simulink library "tp333079"  (Simulink 5.0)
values from neighbouring files (symbols this model uses):
  b = 1    [main_flock3.m]    (also in main_flock4.m; params_flocking_ros.m)
undefined symbols (not defined in the file or in its folder): AC, AlphaBnd, BetaBnd, CDda, CDde, CDdf, CDdr, CDM, CDmin, CGempty, CGgross, CL0, CLa, CLalphadot, Clbeta, Clda, CLde, CLdf, Cldr, CLM, CLmind, Clp, CLq, Clr, Cm0, Cma, Cmalphadot, Cmde, Cmdf, CmM, Cmq, Cnbeta, Cnda, Cndr, Cnp, Cnr, CP, CT, CYbeta, CYda, CYdr, CYp, CYr, Displacement, dmy, Engine, EulerIni, FuelFlow, FuelIni, J, Jempty, Jeng, Jgross, Jprop, MAC, MAP, MAPLim, MassIni, MaxPower, mempty ... (+26)
libraries: aerosimlib x325, simulink3 x42
(part 11 of 11)

== system tp333079/FlightGear-Compatible/Complete Aircraft/CESSNA-172/Aerodynamics/Roll/Cl aileron ==
  RowParam : Inport  Port=1  PortDimensions=-1  SampleTime=-1  DataType=auto
      settings: SignalType=auto
  ColParam : Inport  Port=2  PortDimensions=-1  SampleTime=-1  DataType=auto
      settings: SignalType=auto
  Value : aerosimlib/FlightGear-Compatible/Aerodynamics/Value  Value=AC.Aerodynamics.Roll.ClDa
  term2 : Terminator
  Coeff : Outport  Port=1
  wires:
  RowParam/1 -> Value/1
  Value/1 -> Coeff/1
  ColParam/1 -> term2/1

== system tp333079/FlightGear-Compatible/Complete Aircraft/CESSNA-172/Aerodynamics/Roll/Cl beta ==
  RowParam : Inport  Port=1  PortDimensions=-1  SampleTime=-1  DataType=auto
      settings: SignalType=auto
  ColParam : Inport  Port=2  PortDimensions=-1  SampleTime=-1  DataType=auto
      settings: SignalType=auto
  Vector : aerosimlib/FlightGear-Compatible/Aerodynamics/Vector  Vector=AC.Aerodynamics.Roll.Clb
  term2 : Terminator
  Coeff : Outport  Port=1
  wires:
  RowParam/1 -> Vector/1
  Vector/1 -> Coeff/1
  ColParam/1 -> term2/1

== system tp333079/FlightGear-Compatible/Complete Aircraft/CESSNA-172/Aerodynamics/Roll/Cl rudder ==
  RowParam : Inport  Port=1  PortDimensions=-1  SampleTime=-1  DataType=auto
      settings: SignalType=auto
  ColParam : Inport  Port=2  PortDimensions=-1  SampleTime=-1  DataType=auto
      settings: SignalType=auto
  Value : aerosimlib/FlightGear-Compatible/Aerodynamics/Value  Value=AC.Aerodynamics.Roll.Cldr
  term2 : Terminator
  Coeff : Outport  Port=1
  wires:
  RowParam/1 -> Value/1
  Value/1 -> Coeff/1
  ColParam/1 -> term2/1

== system tp333079/FlightGear-Compatible/Complete Aircraft/CESSNA-172/Aerodynamics/Roll/Clp ==
  RowParam : Inport  Port=1  PortDimensions=-1  SampleTime=-1  DataType=auto
      settings: SignalType=auto
  ColParam : Inport  Port=2  PortDimensions=-1  SampleTime=-1  DataType=auto
      settings: SignalType=auto
  Value : aerosimlib/FlightGear-Compatible/Aerodynamics/Value  Value=AC.Aerodynamics.Roll.Clp
  term2 : Terminator
  Coeff : Outport  Port=1
  wires:
  RowParam/1 -> Value/1
  Value/1 -> Coeff/1
  ColParam/1 -> term2/1

== system tp333079/FlightGear-Compatible/Complete Aircraft/CESSNA-172/Aerodynamics/Roll/Clr ==
  RowParam : Inport  Port=1  PortDimensions=-1  SampleTime=-1  DataType=auto
      settings: SignalType=auto
  ColParam : Inport  Port=2  PortDimensions=-1  SampleTime=-1  DataType=auto
      settings: SignalType=auto
  Table : aerosimlib/FlightGear-Compatible/Aerodynamics/Table  Table=AC.Aerodynamics.Roll.Clr
  Coeff : Outport  Port=1
  wires:
  RowParam/1 -> Table/1
  ColParam/1 -> Table/2
  Table/1 -> Coeff/1

== system tp333079/FlightGear-Compatible/Complete Aircraft/CESSNA-172/Aerodynamics/Side/CY aileron ==
  RowParam : Inport  Port=1  PortDimensions=-1  SampleTime=-1  DataType=auto
      settings: SignalType=auto
  ColParam : Inport  Port=2  PortDimensions=-1  SampleTime=-1  DataType=auto
      settings: SignalType=auto
  Value : aerosimlib/FlightGear-Compatible/Aerodynamics/Value  Value=AC.Aerodynamics.Side.CYda
  term2 : Terminator
  Coeff : Outport  Port=1
  wires:
  RowParam/1 -> Value/1
  Value/1 -> Coeff/1
  ColParam/1 -> term2/1

== system tp333079/FlightGear-Compatible/Complete Aircraft/CESSNA-172/Aerodynamics/Side/CY beta ==
  RowParam : Inport  Port=1  PortDimensions=-1  SampleTime=-1  DataType=auto
      settings: SignalType=auto
  ColParam : Inport  Port=2  PortDimensions=-1  SampleTime=-1  DataType=auto
      settings: SignalType=auto
  Table : aerosimlib/FlightGear-Compatible/Aerodynamics/Table  Table=AC.Aerodynamics.Side.CYb
  Coeff : Outport  Port=1
  wires:
  RowParam/1 -> Table/1
  ColParam/1 -> Table/2
  Table/1 -> Coeff/1

== system tp333079/FlightGear-Compatible/Complete Aircraft/CESSNA-172/Aerodynamics/Side/CY rudder ==
  RowParam : Inport  Port=1  PortDimensions=-1  SampleTime=-1  DataType=auto
      settings: SignalType=auto
  ColParam : Inport  Port=2  PortDimensions=-1  SampleTime=-1  DataType=auto
      settings: SignalType=auto
  Value : aerosimlib/FlightGear-Compatible/Aerodynamics/Value  Value=AC.Aerodynamics.Side.CYdr
  term2 : Terminator
  Coeff : Outport  Port=1
  wires:
  RowParam/1 -> Value/1
  Value/1 -> Coeff/1
  ColParam/1 -> term2/1

== system tp333079/FlightGear-Compatible/Complete Aircraft/CESSNA-172/Aerodynamics/Side/CYp ==
  RowParam : Inport  Port=1  PortDimensions=-1  SampleTime=-1  DataType=auto
      settings: SignalType=auto
  ColParam : Inport  Port=2  PortDimensions=-1  SampleTime=-1  DataType=auto
      settings: SignalType=auto
  Table : aerosimlib/FlightGear-Compatible/Aerodynamics/Table  Table=AC.Aerodynamics.Side.CYp
  Coeff : Outport  Port=1
  wires:
  RowParam/1 -> Table/1
  ColParam/1 -> Table/2
  Table/1 -> Coeff/1

== system tp333079/FlightGear-Compatible/Complete Aircraft/CESSNA-172/Aerodynamics/Side/CYr ==
  RowParam : Inport  Port=1  PortDimensions=-1  SampleTime=-1  DataType=auto
      settings: SignalType=auto
  ColParam : Inport  Port=2  PortDimensions=-1  SampleTime=-1  DataType=auto
      settings: SignalType=auto
  Table : aerosimlib/FlightGear-Compatible/Aerodynamics/Table  Table=AC.Aerodynamics.Side.CYr
  Coeff : Outport  Port=1
  wires:
  RowParam/1 -> Table/1
  ColParam/1 -> Table/2
  Table/1 -> Coeff/1

== system tp333079/FlightGear-Compatible/Complete Aircraft/CESSNA-172/Aerodynamics/Yaw/Cn aileron ==
  RowParam : Inport  Port=1  PortDimensions=-1  SampleTime=-1  DataType=auto
      settings: SignalType=auto
  ColParam : Inport  Port=2  PortDimensions=-1  SampleTime=-1  DataType=auto
      settings: SignalType=auto
  Value : aerosimlib/FlightGear-Compatible/Aerodynamics/Value  Value=AC.Aerodynamics.Yaw.Cnda
  term2 : Terminator
  Coeff : Outport  Port=1
  wires:
  ColParam/1 -> term2/1
  Value/1 -> Coeff/1
  RowParam/1 -> Value/1

== system tp333079/FlightGear-Compatible/Complete Aircraft/CESSNA-172/Aerodynamics/Yaw/Cn beta ==
  RowParam : Inport  Port=1  PortDimensions=-1  SampleTime=-1  DataType=auto
      settings: SignalType=auto
  ColParam : Inport  Port=2  PortDimensions=-1  SampleTime=-1  DataType=auto
      settings: SignalType=auto
  Vector : aerosimlib/FlightGear-Compatible/Aerodynamics/Vector  Vector=AC.Aerodynamics.Yaw.Cnb
  term2 : Terminator
  Coeff : Outport  Port=1
  wires:
  ColParam/1 -> term2/1
  Vector/1 -> Coeff/1
  RowParam/1 -> Vector/1

== system tp333079/FlightGear-Compatible/Complete Aircraft/CESSNA-172/Aerodynamics/Yaw/Cn rudder ==
  RowParam : Inport  Port=1  PortDimensions=-1  SampleTime=-1  DataType=auto
      settings: SignalType=auto
  ColParam : Inport  Port=2  PortDimensions=-1  SampleTime=-1  DataType=auto
      settings: SignalType=auto
  Value : aerosimlib/FlightGear-Compatible/Aerodynamics/Value  Value=AC.Aerodynamics.Yaw.Cndr
  term2 : Terminator
  Coeff : Outport  Port=1
  wires:
  ColParam/1 -> term2/1
  Value/1 -> Coeff/1
  RowParam/1 -> Value/1

== system tp333079/FlightGear-Compatible/Complete Aircraft/CESSNA-172/Aerodynamics/Yaw/Cnp ==
  RowParam : Inport  Port=1  PortDimensions=-1  SampleTime=-1  DataType=auto
      settings: SignalType=auto
  ColParam : Inport  Port=2  PortDimensions=-1  SampleTime=-1  DataType=auto
      settings: SignalType=auto
  Value : aerosimlib/FlightGear-Compatible/Aerodynamics/Value  Value=AC.Aerodynamics.Yaw.Cnp
  term2 : Terminator
  Coeff : Outport  Port=1
  wires:
  ColParam/1 -> term2/1
  Value/1 -> Coeff/1
  RowParam/1 -> Value/1

== system tp333079/FlightGear-Compatible/Complete Aircraft/CESSNA-172/Aerodynamics/Yaw/Cnr ==
  RowParam : Inport  Port=1  PortDimensions=-1  SampleTime=-1  DataType=auto
      settings: SignalType=auto
  ColParam : Inport  Port=2  PortDimensions=-1  SampleTime=-1  DataType=auto
      settings: SignalType=auto
  Value : aerosimlib/FlightGear-Compatible/Aerodynamics/Value  Value=AC.Aerodynamics.Yaw.Cnr
  term2 : Terminator
  Coeff : Outport  Port=1
  wires:
  ColParam/1 -> term2/1
  Value/1 -> Coeff/1
  RowParam/1 -> Value/1

== system tp333079/FlightGear-Compatible/Complete Aircraft/CESSNA-182/Aerodynamics/Drag/CD alpha ==
  RowParam : Inport  Port=1  PortDimensions=-1  SampleTime=-1  DataType=auto
      settings: SignalType=auto
  ColParam : Inport  Port=2  PortDimensions=-1  SampleTime=-1  DataType=auto
      settings: SignalType=auto
  Vector : aerosimlib/FlightGear-Compatible/Aerodynamics/Vector  Vector=AC.Aerodynamics.Drag.CDalpha
  term2 : Terminator
  Coeff : Outport  Port=1
  wires:
  ColParam/1 -> term2/1
  Vector/1 -> Coeff/1
  RowParam/1 -> Vector/1

== system tp333079/FlightGear-Compatible/Complete Aircraft/CESSNA-182/Aerodynamics/Drag/CD beta ==
  RowParam : Inport  Port=1  PortDimensions=-1  SampleTime=-1  DataType=auto
      settings: SignalType=auto
  ColParam : Inport  Port=2  PortDimensions=-1  SampleTime=-1  DataType=auto
      settings: SignalType=auto
  Value : aerosimlib/FlightGear-Compatible/Aerodynamics/Value  Value=AC.Aerodynamics.Drag.CDbeta
  term2 : Terminator
  Coeff : Outport  Port=1
  wires:
  ColParam/1 -> term2/1
  Value/1 -> Coeff/1
  RowParam/1 -> Value/1

== system tp333079/FlightGear-Compatible/Complete Aircraft/CESSNA-182/Aerodynamics/Drag/CD elevator ==
  RowParam : Inport  Port=1  PortDimensions=-1  SampleTime=-1  DataType=auto
      settings: SignalType=auto
  ColParam : Inport  Port=2  PortDimensions=-1  SampleTime=-1  DataType=auto
      settings: SignalType=auto
  Value : aerosimlib/FlightGear-Compatible/Aerodynamics/Value  Value=AC.Aerodynamics.Drag.CDDe
  term2 : Terminator
  Coeff : Outport  Port=1
  wires:
  ColParam/1 -> term2/1
  Value/1 -> Coeff/1
  RowParam/1 -> Value/1

== system tp333079/FlightGear-Compatible/Complete Aircraft/CESSNA-182/Aerodynamics/Drag/CD flap ==
  RowParam : Inport  Port=1  PortDimensions=-1  SampleTime=-1  DataType=auto
      settings: SignalType=auto
  ColParam : Inport  Port=2  PortDimensions=-1  SampleTime=-1  DataType=auto
      settings: SignalType=auto
  Table : aerosimlib/FlightGear-Compatible/Aerodynamics/Table  Table=AC.Aerodynamics.Drag.CDDf
  Coeff : Outport  Port=1
  wires:
  Table/1 -> Coeff/1
  ColParam/1 -> Table/2
  RowParam/1 -> Table/1

== system tp333079/FlightGear-Compatible/Complete Aircraft/CESSNA-182/Aerodynamics/Lift/CL alpha ==
  RowParam : Inport  Port=1  PortDimensions=-1  SampleTime=-1  DataType=auto
      settings: SignalType=auto
  ColParam : Inport  Port=2  PortDimensions=-1  SampleTime=-1  DataType=auto
      settings: SignalType=auto
  Vector : aerosimlib/FlightGear-Compatible/Aerodynamics/Vector  Vector=AC.Aerodynamics.Lift.Basic.CLalpha
  term2 : Terminator
  Coeff : Outport  Port=1
  wires:
  ColParam/1 -> term2/1
  Vector/1 -> Coeff/1
  RowParam/1 -> Vector/1

== system tp333079/FlightGear-Compatible/Complete Aircraft/CESSNA-182/Aerodynamics/Lift/CL elevator ==
  RowParam : Inport  Port=1  PortDimensions=-1  SampleTime=-1  DataType=auto
      settings: SignalType=auto
  ColParam : Inport  Port=2  PortDimensions=-1  SampleTime=-1  DataType=auto
      settings: SignalType=auto
  Value : aerosimlib/FlightGear-Compatible/Aerodynamics/Value  Value=AC.Aerodynamics.Lift.CLDe
  term2 : Terminator
  Coeff : Outport  Port=1
  wires:
  ColParam/1 -> term2/1
  Value/1 -> Coeff/1
  RowParam/1 -> Value/1

== system tp333079/FlightGear-Compatible/Complete Aircraft/CESSNA-182/Aerodynamics/Lift/CL flap ==
  RowParam : Inport  Port=1  PortDimensions=-1  SampleTime=-1  DataType=auto
      settings: SignalType=auto
  ColParam : Inport  Port=2  PortDimensions=-1  SampleTime=-1  DataType=auto
      settings: SignalType=auto
  Vector : aerosimlib/FlightGear-Compatible/Aerodynamics/Vector  Vector=AC.Aerodynamics.Lift.Basic.CLDf
  term2 : Terminator
  Coeff : Outport  Port=1
  wires:
  ColParam/1 -> term2/1
  Vector/1 -> Coeff/1
  RowParam/1 -> Vector/1

== system tp333079/FlightGear-Compatible/Complete Aircraft/CESSNA-182/Aerodynamics/Lift/CLalphadot ==
  RowParam : Inport  Port=1  PortDimensions=-1  SampleTime=-1  DataType=auto
      settings: SignalType=auto
  ColParam : Inport  Port=2  PortDimensions=-1  SampleTime=-1  DataType=auto
      settings: SignalType=auto
  Value : aerosimlib/FlightGear-Compatible/Aerodynamics/Value  Value=AC.Aerodynamics.Lift.CLadot
  term2 : Terminator
  Coeff : Outport  Port=1
  wires:
  ColParam/1 -> term2/1
  Value/1 -> Coeff/1
  RowParam/1 -> Value/1

== system tp333079/FlightGear-Compatible/Complete Aircraft/CESSNA-182/Aerodynamics/Lift/CLq ==
  RowParam : Inport  Port=1  PortDimensions=-1  SampleTime=-1  DataType=auto
      settings: SignalType=auto
  ColParam : Inport  Port=2  PortDimensions=-1  SampleTime=-1  DataType=auto
      settings: SignalType=auto
  Value : aerosimlib/FlightGear-Compatible/Aerodynamics/Value  Value=AC.Aerodynamics.Lift.CLq
  term2 : Terminator
  Coeff : Outport  Port=1
  wires:
  ColParam/1 -> term2/1
  Value/1 -> Coeff/1
  RowParam/1 -> Value/1

== system tp333079/FlightGear-Compatible/Complete Aircraft/CESSNA-182/Aerodynamics/Lift/kCL ground effect ==
  RowParam : Inport  Port=1  PortDimensions=-1  SampleTime=-1  DataType=auto
      settings: SignalType=auto
  ColParam : Inport  Port=2  PortDimensions=-1  SampleTime=-1  DataType=auto
      settings: SignalType=auto
  Vector : aerosimlib/FlightGear-Compatible/Aerodynamics/Vector  Vector=AC.Aerodynamics.Lift.Basic.kCLge
  term2 : Terminator
  Coeff : Outport  Port=1
  wires:
  ColParam/1 -> term2/1
  Vector/1 -> Coeff/1
  RowParam/1 -> Vector/1

== system tp333079/FlightGear-Compatible/Complete Aircraft/CESSNA-182/Aerodynamics/Pitch/Cm alpha ==
  RowParam : Inport  Port=1  PortDimensions=-1  SampleTime=-1  DataType=auto
      settings: SignalType=auto
  ColParam : Inport  Port=2  PortDimensions=-1  SampleTime=-1  DataType=auto
      settings: SignalType=auto
  Vector : aerosimlib/FlightGear-Compatible/Aerodynamics/Vector  Vector=AC.Aerodynamics.Pitch.Cmalpha
  term2 : Terminator
  Coeff : Outport  Port=1
  wires:
  ColParam/1 -> term2/1
  Vector/1 -> Coeff/1
  RowParam/1 -> Vector/1

== system tp333079/FlightGear-Compatible/Complete Aircraft/CESSNA-182/Aerodynamics/Pitch/Cm elevator ==
  RowParam : Inport  Port=1  PortDimensions=-1  SampleTime=-1  DataType=auto
      settings: SignalType=auto
  ColParam : Inport  Port=2  PortDimensions=-1  SampleTime=-1  DataType=auto
      settings: SignalType=auto
  Vector : aerosimlib/FlightGear-Compatible/Aerodynamics/Vector  Vector=AC.Aerodynamics.Pitch.CmDe
  term2 : Terminator
  Coeff : Outport  Port=1
  wires:
  ColParam/1 -> term2/1
  Vector/1 -> Coeff/1
  RowParam/1 -> Vector/1

== system tp333079/FlightGear-Compatible/Complete Aircraft/CESSNA-182/Aerodynamics/Pitch/Cm flap ==
  RowParam : Inport  Port=1  PortDimensions=-1  SampleTime=-1  DataType=auto
      settings: SignalType=auto
  ColParam : Inport  Port=2  PortDimensions=-1  SampleTime=-1  DataType=auto
      settings: SignalType=auto
  Vector : aerosimlib/FlightGear-Compatible/Aerodynamics/Vector  Vector=AC.Aerodynamics.Pitch.CmDf
  term2 : Terminator
  Coeff : Outport  Port=1
  wires:
  ColParam/1 -> term2/1
  Vector/1 -> Coeff/1
  RowParam/1 -> Vector/1

== system tp333079/FlightGear-Compatible/Complete Aircraft/CESSNA-182/Aerodynamics/Pitch/Cmalphadot ==
  RowParam : Inport  Port=1  PortDimensions=-1  SampleTime=-1  DataType=auto
      settings: SignalType=auto
  ColParam : Inport  Port=2  PortDimensions=-1  SampleTime=-1  DataType=auto
      settings: SignalType=auto
  Vector : aerosimlib/FlightGear-Compatible/Aerodynamics/Vector  Vector=AC.Aerodynamics.Pitch.Cmadot
  term2 : Terminator
  Coeff : Outport  Port=1
  wires:
  ColParam/1 -> term2/1
  Vector/1 -> Coeff/1
  RowParam/1 -> Vector/1

== system tp333079/FlightGear-Compatible/Complete Aircraft/CESSNA-182/Aerodynamics/Pitch/Cmq ==
  RowParam : Inport  Port=1  PortDimensions=-1  SampleTime=-1  DataType=auto
      settings: SignalType=auto
  ColParam : Inport  Port=2  PortDimensions=-1  SampleTime=-1  DataType=auto
      settings: SignalType=auto
  Value : aerosimlib/FlightGear-Compatible/Aerodynamics/Value  Value=AC.Aerodynamics.Pitch.Cmq
  term2 : Terminator
  Coeff : Outport  Port=1
  wires:
  ColParam/1 -> term2/1
  Value/1 -> Coeff/1
  RowParam/1 -> Value/1

== system tp333079/FlightGear-Compatible/Complete Aircraft/CESSNA-182/Aerodynamics/Roll/Cl aileron ==
  RowParam : Inport  Port=1  PortDimensions=-1  SampleTime=-1  DataType=auto
      settings: SignalType=auto
  ColParam : Inport  Port=2  PortDimensions=-1  SampleTime=-1  DataType=auto
      settings: SignalType=auto
  Value : aerosimlib/FlightGear-Compatible/Aerodynamics/Value  Value=AC.Aerodynamics.Roll.ClDa
  term2 : Terminator
  Coeff : Outport  Port=1
  wires:
  ColParam/1 -> term2/1
  Value/1 -> Coeff/1
  RowParam/1 -> Value/1

== system tp333079/FlightGear-Compatible/Complete Aircraft/CESSNA-182/Aerodynamics/Roll/Cl beta ==
  RowParam : Inport  Port=1  PortDimensions=-1  SampleTime=-1  DataType=auto
      settings: SignalType=auto
  ColParam : Inport  Port=2  PortDimensions=-1  SampleTime=-1  DataType=auto
      settings: SignalType=auto
  Table : aerosimlib/FlightGear-Compatible/Aerodynamics/Table  Table=AC.Aerodynamics.Roll.Clb
  Coeff : Outport  Port=1
  wires:
  Table/1 -> Coeff/1
  ColParam/1 -> Table/2
  RowParam/1 -> Table/1

== system tp333079/FlightGear-Compatible/Complete Aircraft/CESSNA-182/Aerodynamics/Roll/Cl rudder ==
  RowParam : Inport  Port=1  PortDimensions=-1  SampleTime=-1  DataType=auto
      settings: SignalType=auto
  ColParam : Inport  Port=2  PortDimensions=-1  SampleTime=-1  DataType=auto
      settings: SignalType=auto
  Value : aerosimlib/FlightGear-Compatible/Aerodynamics/Value  Value=AC.Aerodynamics.Roll.ClDr
  term2 : Terminator
  Coeff : Outport  Port=1
  wires:
  ColParam/1 -> term2/1
  Value/1 -> Coeff/1
  RowParam/1 -> Value/1

== system tp333079/FlightGear-Compatible/Complete Aircraft/CESSNA-182/Aerodynamics/Roll/Clp ==
  RowParam : Inport  Port=1  PortDimensions=-1  SampleTime=-1  DataType=auto
      settings: SignalType=auto
  ColParam : Inport  Port=2  PortDimensions=-1  SampleTime=-1  DataType=auto
      settings: SignalType=auto
  Vector : aerosimlib/FlightGear-Compatible/Aerodynamics/Vector  Vector=AC.Aerodynamics.Roll.Clp
  term2 : Terminator
  Coeff : Outport  Port=1
  wires:
  ColParam/1 -> term2/1
  Vector/1 -> Coeff/1
  RowParam/1 -> Vector/1

== system tp333079/FlightGear-Compatible/Complete Aircraft/CESSNA-182/Aerodynamics/Roll/Clr ==
  RowParam : Inport  Port=1  PortDimensions=-1  SampleTime=-1  DataType=auto
      settings: SignalType=auto
  ColParam : Inport  Port=2  PortDimensions=-1  SampleTime=-1  DataType=auto
      settings: SignalType=auto
  Vector : aerosimlib/FlightGear-Compatible/Aerodynamics/Vector  Vector=AC.Aerodynamics.Roll.Clr
  term2 : Terminator
  Coeff : Outport  Port=1
  wires:
  ColParam/1 -> term2/1
  Vector/1 -> Coeff/1
  RowParam/1 -> Vector/1

== system tp333079/FlightGear-Compatible/Complete Aircraft/CESSNA-182/Aerodynamics/Side/CY aileron ==
  RowParam : Inport  Port=1  PortDimensions=-1  SampleTime=-1  DataType=auto
      settings: SignalType=auto
  ColParam : Inport  Port=2  PortDimensions=-1  SampleTime=-1  DataType=auto
      settings: SignalType=auto
  Value : aerosimlib/FlightGear-Compatible/Aerodynamics/Value  Value=AC.Aerodynamics.Side.CYDa
  term2 : Terminator
  Coeff : Outport  Port=1
  wires:
  ColParam/1 -> term2/1
  Value/1 -> Coeff/1
  RowParam/1 -> Value/1

== system tp333079/FlightGear-Compatible/Complete Aircraft/CESSNA-182/Aerodynamics/Side/CY beta ==
  RowParam : Inport  Port=1  PortDimensions=-1  SampleTime=-1  DataType=auto
      settings: SignalType=auto
  ColParam : Inport  Port=2  PortDimensions=-1  SampleTime=-1  DataType=auto
      settings: SignalType=auto
  Vector : aerosimlib/FlightGear-Compatible/Aerodynamics/Vector  Vector=AC.Aerodynamics.Side.CYb
  term2 : Terminator
  Coeff : Outport  Port=1
  wires:
  ColParam/1 -> term2/1
  Vector/1 -> Coeff/1
  RowParam/1 -> Vector/1

== system tp333079/FlightGear-Compatible/Complete Aircraft/CESSNA-182/Aerodynamics/Side/CY rudder ==
  RowParam : Inport  Port=1  PortDimensions=-1  SampleTime=-1  DataType=auto
      settings: SignalType=auto
  ColParam : Inport  Port=2  PortDimensions=-1  SampleTime=-1  DataType=auto
      settings: SignalType=auto
  Value : aerosimlib/FlightGear-Compatible/Aerodynamics/Value  Value=AC.Aerodynamics.Side.CYDr
  term2 : Terminator
  Coeff : Outport  Port=1
  wires:
  ColParam/1 -> term2/1
  Value/1 -> Coeff/1
  RowParam/1 -> Value/1

== system tp333079/FlightGear-Compatible/Complete Aircraft/CESSNA-182/Aerodynamics/Side/CYp ==
  RowParam : Inport  Port=1  PortDimensions=-1  SampleTime=-1  DataType=auto
      settings: SignalType=auto
  ColParam : Inport  Port=2  PortDimensions=-1  SampleTime=-1  DataType=auto
      settings: SignalType=auto
  Vector : aerosimlib/FlightGear-Compatible/Aerodynamics/Vector  Vector=AC.Aerodynamics.Side.CYp
  term2 : Terminator
  Coeff : Outport  Port=1
  wires:
  ColParam/1 -> term2/1
  Vector/1 -> Coeff/1
  RowParam/1 -> Vector/1

== system tp333079/FlightGear-Compatible/Complete Aircraft/CESSNA-182/Aerodynamics/Side/CYr ==
  RowParam : Inport  Port=1  PortDimensions=-1  SampleTime=-1  DataType=auto
      settings: SignalType=auto
  ColParam : Inport  Port=2  PortDimensions=-1  SampleTime=-1  DataType=auto
      settings: SignalType=auto
  Vector : aerosimlib/FlightGear-Compatible/Aerodynamics/Vector  Vector=AC.Aerodynamics.Side.CYr
  term2 : Terminator
  Coeff : Outport  Port=1
  wires:
  ColParam/1 -> term2/1
  Vector/1 -> Coeff/1
  RowParam/1 -> Vector/1

== system tp333079/FlightGear-Compatible/Complete Aircraft/CESSNA-182/Aerodynamics/Yaw/Cn aileron ==
  RowParam : Inport  Port=1  PortDimensions=-1  SampleTime=-1  DataType=auto
      settings: SignalType=auto
  ColParam : Inport  Port=2  PortDimensions=-1  SampleTime=-1  DataType=auto
      settings: SignalType=auto
  Vector : aerosimlib/FlightGear-Compatible/Aerodynamics/Vector  Vector=AC.Aerodynamics.Yaw.CnDa
  term2 : Terminator
  Coeff : Outport  Port=1
  wires:
  ColParam/1 -> term2/1
  Vector/1 -> Coeff/1
  RowParam/1 -> Vector/1

== system tp333079/FlightGear-Compatible/Complete Aircraft/CESSNA-182/Aerodynamics/Yaw/Cn beta ==
  RowParam : Inport  Port=1  PortDimensions=-1  SampleTime=-1  DataType=auto
      settings: SignalType=auto
  ColParam : Inport  Port=2  PortDimensions=-1  SampleTime=-1  DataType=auto
      settings: SignalType=auto
  Vector : aerosimlib/FlightGear-Compatible/Aerodynamics/Vector  Vector=AC.Aerodynamics.Yaw.Cnb
  term2 : Terminator
  Coeff : Outport  Port=1
  wires:
  ColParam/1 -> term2/1
  Vector/1 -> Coeff/1
  RowParam/1 -> Vector/1

== system tp333079/FlightGear-Compatible/Complete Aircraft/CESSNA-182/Aerodynamics/Yaw/Cn rudder ==
  RowParam : Inport  Port=1  PortDimensions=-1  SampleTime=-1  DataType=auto
      settings: SignalType=auto
  ColParam : Inport  Port=2  PortDimensions=-1  SampleTime=-1  DataType=auto
      settings: SignalType=auto
  Vector : aerosimlib/FlightGear-Compatible/Aerodynamics/Vector  Vector=AC.Aerodynamics.Yaw.CnDr
  term2 : Terminator
  Coeff : Outport  Port=1
  wires:
  ColParam/1 -> term2/1
  Vector/1 -> Coeff/1
  RowParam/1 -> Vector/1

== system tp333079/FlightGear-Compatible/Complete Aircraft/CESSNA-182/Aerodynamics/Yaw/Cnp ==
  RowParam : Inport  Port=1  PortDimensions=-1  SampleTime=-1  DataType=auto
      settings: SignalType=auto
  ColParam : Inport  Port=2  PortDimensions=-1  SampleTime=-1  DataType=auto
      settings: SignalType=auto
  Vector : aerosimlib/FlightGear-Compatible/Aerodynamics/Vector  Vector=AC.Aerodynamics.Yaw.Cnp
  term2 : Terminator
  Coeff : Outport  Port=1
  wires:
  ColParam/1 -> term2/1
  Vector/1 -> Coeff/1
  RowParam/1 -> Vector/1

== system tp333079/FlightGear-Compatible/Complete Aircraft/CESSNA-182/Aerodynamics/Yaw/Cnr ==
  RowParam : Inport  Port=1  PortDimensions=-1  SampleTime=-1  DataType=auto
      settings: SignalType=auto
  ColParam : Inport  Port=2  PortDimensions=-1  SampleTime=-1  DataType=auto
      settings: SignalType=auto
  Vector : aerosimlib/FlightGear-Compatible/Aerodynamics/Vector  Vector=AC.Aerodynamics.Yaw.Cnr
  term2 : Terminator
  Coeff : Outport  Port=1
  wires:
  ColParam/1 -> term2/1
  Vector/1 -> Coeff/1
  RowParam/1 -> Vector/1

== system tp333079/FlightGear-Compatible/Complete Aircraft/CESSNA-310/Aerodynamics/Drag/CD alpha ==
  RowParam : Inport  Port=1  PortDimensions=-1  SampleTime=-1  DataType=auto
      settings: SignalType=auto
  ColParam : Inport  Port=2  PortDimensions=-1  SampleTime=-1  DataType=auto
      settings: SignalType=auto
  Vector : aerosimlib/FlightGear-Compatible/Aerodynamics/Vector  Vector=AC.Aerodynamics.Drag.CDalpha
  term2 : Terminator
  Coeff : Outport  Port=1
  wires:
  RowParam/1 -> Vector/1
  Vector/1 -> Coeff/1
  ColParam/1 -> term2/1

== system tp333079/FlightGear-Compatible/Complete Aircraft/CESSNA-310/Aerodynamics/Drag/CD beta ==
  RowParam : Inport  Port=1  PortDimensions=-1  SampleTime=-1  DataType=auto
      settings: SignalType=auto
  ColParam : Inport  Port=2  PortDimensions=-1  SampleTime=-1  DataType=auto
      settings: SignalType=auto
  Value : aerosimlib/FlightGear-Compatible/Aerodynamics/Value  Value=AC.Aerodynamics.Drag.CDbeta
  term2 : Terminator
  Coeff : Outport  Port=1
  wires:
  RowParam/1 -> Value/1
  Value/1 -> Coeff/1
  ColParam/1 -> term2/1

== system tp333079/FlightGear-Compatible/Complete Aircraft/CESSNA-310/Aerodynamics/Drag/CD elevator ==
  RowParam : Inport  Port=1  PortDimensions=-1  SampleTime=-1  DataType=auto
      settings: SignalType=auto
  ColParam : Inport  Port=2  PortDimensions=-1  SampleTime=-1  DataType=auto
      settings: SignalType=auto
  Value : aerosimlib/FlightGear-Compatible/Aerodynamics/Value  Value=AC.Aerodynamics.Drag.CDDe
  term2 : Terminator
  Coeff : Outport  Port=1
  wires:
  RowParam/1 -> Value/1
  Value/1 -> Coeff/1
  ColParam/1 -> term2/1

== system tp333079/FlightGear-Compatible/Complete Aircraft/CESSNA-310/Aerodynamics/Drag/CD flap ==
  RowParam : Inport  Port=1  PortDimensions=-1  SampleTime=-1  DataType=auto
      settings: SignalType=auto
  ColParam : Inport  Port=2  PortDimensions=-1  SampleTime=-1  DataType=auto
      settings: SignalType=auto
  Vector : aerosimlib/FlightGear-Compatible/Aerodynamics/Vector  Vector=AC.Aerodynamics.Drag.CDDf
  term2 : Terminator
  Coeff : Outport  Port=1
  wires:
  RowParam/1 -> Vector/1
  Vector/1 -> Coeff/1
  ColParam/1 -> term2/1

== system tp333079/FlightGear-Compatible/Complete Aircraft/CESSNA-310/Aerodynamics/Drag/CD gear ==
  RowParam : Inport  Port=1  PortDimensions=-1  SampleTime=-1  DataType=auto
      settings: SignalType=auto
  ColParam : Inport  Port=2  PortDimensions=-1  SampleTime=-1  DataType=auto
      settings: SignalType=auto
  Value : aerosimlib/FlightGear-Compatible/Aerodynamics/Value  Value=AC.Aerodynamics.Drag.CDgear
  term2 : Terminator
  Coeff : Outport  Port=1
  wires:
  RowParam/1 -> Value/1
  Value/1 -> Coeff/1
  ColParam/1 -> term2/1

== system tp333079/FlightGear-Compatible/Complete Aircraft/CESSNA-310/Aerodynamics/Lift/CL alpha ==
  RowParam : Inport  Port=1  PortDimensions=-1  SampleTime=-1  DataType=auto
      settings: SignalType=auto
  ColParam : Inport  Port=2  PortDimensions=-1  SampleTime=-1  DataType=auto
      settings: SignalType=auto
  Vector : aerosimlib/FlightGear-Compatible/Aerodynamics/Vector  Vector=AC.Aerodynamics.Lift.Basic.CLalpha
  term2 : Terminator
  Coeff : Outport  Port=1
  wires:
  ColParam/1 -> term2/1
  Vector/1 -> Coeff/1
  RowParam/1 -> Vector/1

== system tp333079/FlightGear-Compatible/Complete Aircraft/CESSNA-310/Aerodynamics/Lift/CL elevator ==
  RowParam : Inport  Port=1  PortDimensions=-1  SampleTime=-1  DataType=auto
      settings: SignalType=auto
  ColParam : Inport  Port=2  PortDimensions=-1  SampleTime=-1  DataType=auto
      settings: SignalType=auto
  Vector : aerosimlib/FlightGear-Compatible/Aerodynamics/Vector  Vector=AC.Aerodynamics.Lift.CLDe
  term2 : Terminator
  Coeff : Outport  Port=1
  wires:
  ColParam/1 -> term2/1
  Vector/1 -> Coeff/1
  RowParam/1 -> Vector/1

== system tp333079/FlightGear-Compatible/Complete Aircraft/CESSNA-310/Aerodynamics/Lift/CL flap ==
  RowParam : Inport  Port=1  PortDimensions=-1  SampleTime=-1  DataType=auto
      settings: SignalType=auto
  ColParam : Inport  Port=2  PortDimensions=-1  SampleTime=-1  DataType=auto
      settings: SignalType=auto
  Vector : aerosimlib/FlightGear-Compatible/Aerodynamics/Vector  Vector=AC.Aerodynamics.Lift.Basic.CLDf
  term2 : Terminator
  Coeff : Outport  Port=1
  wires:
  ColParam/1 -> term2/1
  Vector/1 -> Coeff/1
  RowParam/1 -> Vector/1

== system tp333079/FlightGear-Compatible/Complete Aircraft/CESSNA-310/Aerodynamics/Lift/CLalphadot ==
  RowParam : Inport  Port=1  PortDimensions=-1  SampleTime=-1  DataType=auto
      settings: SignalType=auto
  ColParam : Inport  Port=2  PortDimensions=-1  SampleTime=-1  DataType=auto
      settings: SignalType=auto
  Vector : aerosimlib/FlightGear-Compatible/Aerodynamics/Vector  Vector=AC.Aerodynamics.Lift.CLadot
  term2 : Terminator
  Coeff : Outport  Port=1
  wires:
  ColParam/1 -> term2/1
  Vector/1 -> Coeff/1
  RowParam/1 -> Vector/1

== system tp333079/FlightGear-Compatible/Complete Aircraft/CESSNA-310/Aerodynamics/Lift/CLq ==
  RowParam : Inport  Port=1  PortDimensions=-1  SampleTime=-1  DataType=auto
      settings: SignalType=auto
  ColParam : Inport  Port=2  PortDimensions=-1  SampleTime=-1  DataType=auto
      settings: SignalType=auto
  Vector : aerosimlib/FlightGear-Compatible/Aerodynamics/Vector  Vector=AC.Aerodynamics.Lift.CLq
  term2 : Terminator
  Coeff : Outport  Port=1
  wires:
  ColParam/1 -> term2/1
  Vector/1 -> Coeff/1
  RowParam/1 -> Vector/1

== system tp333079/FlightGear-Compatible/Complete Aircraft/CESSNA-310/Aerodynamics/Lift/kCL ground effect ==
  RowParam : Inport  Port=1  PortDimensions=-1  SampleTime=-1  DataType=auto
      settings: SignalType=auto
  ColParam : Inport  Port=2  PortDimensions=-1  SampleTime=-1  DataType=auto
      settings: SignalType=auto
  Vector : aerosimlib/FlightGear-Compatible/Aerodynamics/Vector  Vector=AC.Aerodynamics.Lift.Basic.kCLge
  term2 : Terminator
  Coeff : Outport  Port=1
  wires:
  ColParam/1 -> term2/1
  Vector/1 -> Coeff/1
  RowParam/1 -> Vector/1

== system tp333079/FlightGear-Compatible/Complete Aircraft/CESSNA-310/Aerodynamics/Pitch/Cm alpha ==
  RowParam : Inport  Port=1  PortDimensions=-1  SampleTime=-1  DataType=auto
      settings: SignalType=auto
  ColParam : Inport  Port=2  PortDimensions=-1  SampleTime=-1  DataType=auto
      settings: SignalType=auto
  Value : aerosimlib/FlightGear-Compatible/Aerodynamics/Value  Value=AC.Aerodynamics.Pitch.Cmalpha
  term2 : Terminator
  Coeff : Outport  Port=1
  wires:
  RowParam/1 -> Value/1
  Value/1 -> Coeff/1
  ColParam/1 -> term2/1

== system tp333079/FlightGear-Compatible/Complete Aircraft/CESSNA-310/Aerodynamics/Pitch/Cm elevator ==
  RowParam : Inport  Port=1  PortDimensions=-1  SampleTime=-1  DataType=auto
      settings: SignalType=auto
  ColParam : Inport  Port=2  PortDimensions=-1  SampleTime=-1  DataType=auto
      settings: SignalType=auto
  Value : aerosimlib/FlightGear-Compatible/Aerodynamics/Value  Value=AC.Aerodynamics.Pitch.CmDe
  term2 : Terminator
  Coeff : Outport  Port=1
  wires:
  RowParam/1 -> Value/1
  Value/1 -> Coeff/1
  ColParam/1 -> term2/1

== system tp333079/FlightGear-Compatible/Complete Aircraft/CESSNA-310/Aerodynamics/Pitch/Cm flap ==
  RowParam : Inport  Port=1  PortDimensions=-1  SampleTime=-1  DataType=auto
      settings: SignalType=auto
  ColParam : Inport  Port=2  PortDimensions=-1  SampleTime=-1  DataType=auto
      settings: SignalType=auto
  Vector : aerosimlib/FlightGear-Compatible/Aerodynamics/Vector  Vector=AC.Aerodynamics.Pitch.CmDf
  term2 : Terminator
  Coeff : Outport  Port=1
  wires:
  RowParam/1 -> Vector/1
  Vector/1 -> Coeff/1
  ColParam/1 -> term2/1

== system tp333079/FlightGear-Compatible/Complete Aircraft/CESSNA-310/Aerodynamics/Pitch/Cmalphadot ==
  RowParam : Inport  Port=1  PortDimensions=-1  SampleTime=-1  DataType=auto
      settings: SignalType=auto
  ColParam : Inport  Port=2  PortDimensions=-1  SampleTime=-1  DataType=auto
      settings: SignalType=auto
  Value : aerosimlib/FlightGear-Compatible/Aerodynamics/Value  Value=AC.Aerodynamics.Pitch.Cmadot
  term2 : Terminator
  Coeff : Outport  Port=1
  wires:
  RowParam/1 -> Value/1
  Value/1 -> Coeff/1
  ColParam/1 -> term2/1

== system tp333079/FlightGear-Compatible/Complete Aircraft/CESSNA-310/Aerodynamics/Pitch/Cmq ==
  RowParam : Inport  Port=1  PortDimensions=-1  SampleTime=-1  DataType=auto
      settings: SignalType=auto
  ColParam : Inport  Port=2  PortDimensions=-1  SampleTime=-1  DataType=auto
      settings: SignalType=auto
  Value : aerosimlib/FlightGear-Compatible/Aerodynamics/Value  Value=AC.Aerodynamics.Pitch.Cmq
  term2 : Terminator
  Coeff : Outport  Port=1
  wires:
  RowParam/1 -> Value/1
  Value/1 -> Coeff/1
  ColParam/1 -> term2/1

== system tp333079/FlightGear-Compatible/Complete Aircraft/CESSNA-310/Aerodynamics/Roll/Cl aileron ==
  RowParam : Inport  Port=1  PortDimensions=-1  SampleTime=-1  DataType=auto
      settings: SignalType=auto
  ColParam : Inport  Port=2  PortDimensions=-1  SampleTime=-1  DataType=auto
      settings: SignalType=auto
  Value : aerosimlib/FlightGear-Compatible/Aerodynamics/Value  Value=AC.Aerodynamics.Roll.ClDa
  term2 : Terminator
  Coeff : Outport  Port=1
  wires:
  RowParam/1 -> Value/1
  Value/1 -> Coeff/1
  ColParam/1 -> term2/1

== system tp333079/FlightGear-Compatible/Complete Aircraft/CESSNA-310/Aerodynamics/Roll/Cl beta ==
  RowParam : Inport  Port=1  PortDimensions=-1  SampleTime=-1  DataType=auto
      settings: SignalType=auto
  ColParam : Inport  Port=2  PortDimensions=-1  SampleTime=-1  DataType=auto
      settings: SignalType=auto
  Vector : aerosimlib/FlightGear-Compatible/Aerodynamics/Vector  Vector=AC.Aerodynamics.Roll.Clbeta
  term2 : Terminator
  Coeff : Outport  Port=1
  wires:
  RowParam/1 -> Vector/1
  Vector/1 -> Coeff/1
  ColParam/1 -> term2/1

== system tp333079/FlightGear-Compatible/Complete Aircraft/CESSNA-310/Aerodynamics/Roll/Cl rudder ==
  RowParam : Inport  Port=1  PortDimensions=-1  SampleTime=-1  DataType=auto
      settings: SignalType=auto
  ColParam : Inport  Port=2  PortDimensions=-1  SampleTime=-1  DataType=auto
      settings: SignalType=auto
  Value : aerosimlib/FlightGear-Compatible/Aerodynamics/Value  Value=AC.Aerodynamics.Roll.Cldr
  term2 : Terminator
  Coeff : Outport  Port=1
  wires:
  RowParam/1 -> Value/1
  Value/1 -> Coeff/1
  ColParam/1 -> term2/1

== system tp333079/FlightGear-Compatible/Complete Aircraft/CESSNA-310/Aerodynamics/Roll/Clp ==
  RowParam : Inport  Port=1  PortDimensions=-1  SampleTime=-1  DataType=auto
      settings: SignalType=auto
  ColParam : Inport  Port=2  PortDimensions=-1  SampleTime=-1  DataType=auto
      settings: SignalType=auto
  Value : aerosimlib/FlightGear-Compatible/Aerodynamics/Value  Value=AC.Aerodynamics.Roll.Clp
  term2 : Terminator
  Coeff : Outport  Port=1
  wires:
  RowParam/1 -> Value/1
  Value/1 -> Coeff/1
  ColParam/1 -> term2/1

== system tp333079/FlightGear-Compatible/Complete Aircraft/CESSNA-310/Aerodynamics/Roll/Clr ==
  RowParam : Inport  Port=1  PortDimensions=-1  SampleTime=-1  DataType=auto
      settings: SignalType=auto
  ColParam : Inport  Port=2  PortDimensions=-1  SampleTime=-1  DataType=auto
      settings: SignalType=auto
  Value : aerosimlib/FlightGear-Compatible/Aerodynamics/Value  Value=AC.Aerodynamics.Roll.Clr
  term2 : Terminator
  Coeff : Outport  Port=1
  wires:
  RowParam/1 -> Value/1
  Value/1 -> Coeff/1
  ColParam/1 -> term2/1

== system tp333079/FlightGear-Compatible/Complete Aircraft/CESSNA-310/Aerodynamics/Side/CY beta ==
  RowParam : Inport  Port=1  PortDimensions=-1  SampleTime=-1  DataType=auto
      settings: SignalType=auto
  ColParam : Inport  Port=2  PortDimensions=-1  SampleTime=-1  DataType=auto
      settings: SignalType=auto
  Vector : aerosimlib/FlightGear-Compatible/Aerodynamics/Vector  Vector=AC.Aerodynamics.Side.CYbeta
  term2 : Terminator
  Coeff : Outport  Port=1
  wires:
  RowParam/1 -> Vector/1
  Vector/1 -> Coeff/1
  ColParam/1 -> term2/1

== system tp333079/FlightGear-Compatible/Complete Aircraft/CESSNA-310/Aerodynamics/Side/CY rudder ==
  RowParam : Inport  Port=1  PortDimensions=-1  SampleTime=-1  DataType=auto
      settings: SignalType=auto
  ColParam : Inport  Port=2  PortDimensions=-1  SampleTime=-1  DataType=auto
      settings: SignalType=auto
  Value : aerosimlib/FlightGear-Compatible/Aerodynamics/Value  Value=AC.Aerodynamics.Side.CYDr
  term2 : Terminator
  Coeff : Outport  Port=1
  wires:
  RowParam/1 -> Value/1
  Value/1 -> Coeff/1
  ColParam/1 -> term2/1

== system tp333079/FlightGear-Compatible/Complete Aircraft/CESSNA-310/Aerodynamics/Side/CYp ==
  RowParam : Inport  Port=1  PortDimensions=-1  SampleTime=-1  DataType=auto
      settings: SignalType=auto
  ColParam : Inport  Port=2  PortDimensions=-1  SampleTime=-1  DataType=auto
      settings: SignalType=auto
  Value : aerosimlib/FlightGear-Compatible/Aerodynamics/Value  Value=AC.Aerodynamics.Side.CYp
  term2 : Terminator
  Coeff : Outport  Port=1
  wires:
  RowParam/1 -> Value/1
  Value/1 -> Coeff/1
  ColParam/1 -> term2/1

== system tp333079/FlightGear-Compatible/Complete Aircraft/CESSNA-310/Aerodynamics/Side/CYr ==
  RowParam : Inport  Port=1  PortDimensions=-1  SampleTime=-1  DataType=auto
      settings: SignalType=auto
  ColParam : Inport  Port=2  PortDimensions=-1  SampleTime=-1  DataType=auto
      settings: SignalType=auto
  Value : aerosimlib/FlightGear-Compatible/Aerodynamics/Value  Value=AC.Aerodynamics.Side.CYr
  term2 : Terminator
  Coeff : Outport  Port=1
  wires:
  RowParam/1 -> Value/1
  Value/1 -> Coeff/1
  ColParam/1 -> term2/1

== system tp333079/FlightGear-Compatible/Complete Aircraft/CESSNA-310/Aerodynamics/Yaw/Cn aileron ==
  RowParam : Inport  Port=1  PortDimensions=-1  SampleTime=-1  DataType=auto
      settings: SignalType=auto
  ColParam : Inport  Port=2  PortDimensions=-1  SampleTime=-1  DataType=auto
      settings: SignalType=auto
  Value : aerosimlib/FlightGear-Compatible/Aerodynamics/Value  Value=AC.Aerodynamics.Yaw.CnDa
  term2 : Terminator
  Coeff : Outport  Port=1
  wires:
  RowParam/1 -> Value/1
  Value/1 -> Coeff/1
  ColParam/1 -> term2/1

== system tp333079/FlightGear-Compatible/Complete Aircraft/CESSNA-310/Aerodynamics/Yaw/Cn beta ==
  RowParam : Inport  Port=1  PortDimensions=-1  SampleTime=-1  DataType=auto
      settings: SignalType=auto
  ColParam : Inport  Port=2  PortDimensions=-1  SampleTime=-1  DataType=auto
      settings: SignalType=auto
  Value : aerosimlib/FlightGear-Compatible/Aerodynamics/Value  Value=AC.Aerodynamics.Yaw.Cnbeta
  term2 : Terminator
  Coeff : Outport  Port=1
  wires:
  RowParam/1 -> Value/1
  Value/1 -> Coeff/1
  ColParam/1 -> term2/1

== system tp333079/FlightGear-Compatible/Complete Aircraft/CESSNA-310/Aerodynamics/Yaw/Cn rudder ==
  RowParam : Inport  Port=1  PortDimensions=-1  SampleTime=-1  DataType=auto
      settings: SignalType=auto
  ColParam : Inport  Port=2  PortDimensions=-1  SampleTime=-1  DataType=auto
      settings: SignalType=auto
  Value : aerosimlib/FlightGear-Compatible/Aerodynamics/Value  Value=AC.Aerodynamics.Yaw.CnDr
  term2 : Terminator
  Coeff : Outport  Port=1
  wires:
  RowParam/1 -> Value/1
  Value/1 -> Coeff/1
  ColParam/1 -> term2/1

== system tp333079/FlightGear-Compatible/Complete Aircraft/CESSNA-310/Aerodynamics/Yaw/Cnp ==
  RowParam : Inport  Port=1  PortDimensions=-1  SampleTime=-1  DataType=auto
      settings: SignalType=auto
  ColParam : Inport  Port=2  PortDimensions=-1  SampleTime=-1  DataType=auto
      settings: SignalType=auto
  Value : aerosimlib/FlightGear-Compatible/Aerodynamics/Value  Value=AC.Aerodynamics.Yaw.Cnp
  term2 : Terminator
  Coeff : Outport  Port=1
  wires:
  RowParam/1 -> Value/1
  Value/1 -> Coeff/1
  ColParam/1 -> term2/1

== system tp333079/FlightGear-Compatible/Complete Aircraft/CESSNA-310/Aerodynamics/Yaw/Cnr ==
  RowParam : Inport  Port=1  PortDimensions=-1  SampleTime=-1  DataType=auto
      settings: SignalType=auto
  ColParam : Inport  Port=2  PortDimensions=-1  SampleTime=-1  DataType=auto
      settings: SignalType=auto
  Value : aerosimlib/FlightGear-Compatible/Aerodynamics/Value  Value=AC.Aerodynamics.Yaw.Cnr
  term2 : Terminator
  Coeff : Outport  Port=1
  wires:
  RowParam/1 -> Value/1
  Value/1 -> Coeff/1
  ColParam/1 -> term2/1
